simulink model "Cartpole_simulink"  (R2023a)
settings: Solver=FixedStepAuto  StartTime=0.0  StopTime=20  FixedStep=0.1  RelTol=1e-3
settings Model: Creator=rohan  LastModifiedBy=harsh
settings OptimizationCC: ReuseModelBlockBuffer=off

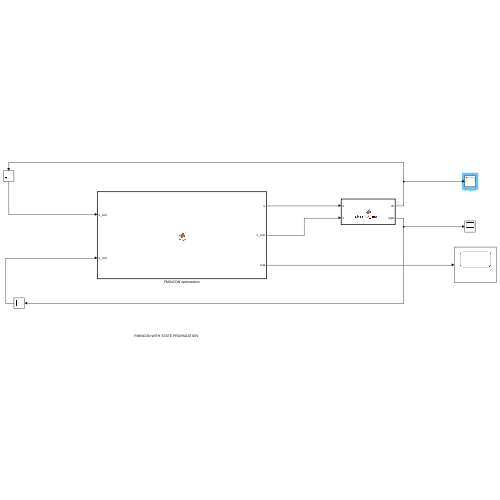
[thumbnail: Simulink's stored preview of the top-level diagram]
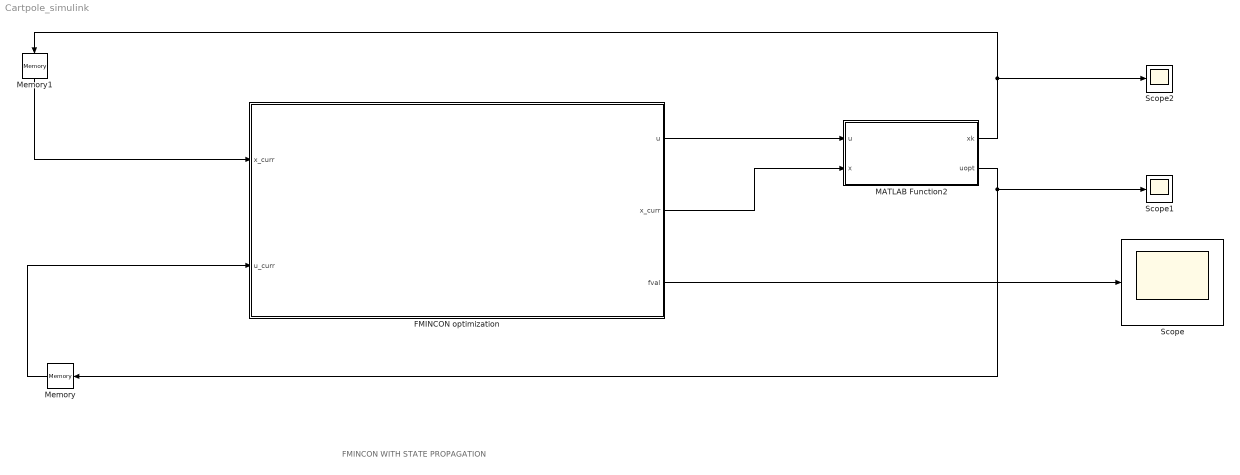
== system Cartpole_simulink ==
  note: FMINCON WITH STATE PROPAGATION
  FMINCON optimization : MATLAB Function  TreatAsAtomicUnit=on
  MATLAB Function2 : MATLAB Function  TreatAsAtomicUnit=on
  Memory : Memory  InitialCondition=zeros(10,1)
  Memory1 : Memory  InitialCondition=[0;0;-pi;0]
  Scope : Scope
  Scope1 : Scope
  Scope2 : Scope
  wires:
  FMINCON optimization/3(fval) -> Scope/1
  Memory/1 -> FMINCON optimization/2(u_curr)
  Memory1/1 -> FMINCON optimization/1("x_curr ")
  FMINCON optimization/1(u) -> MATLAB Function2/1(u)
  FMINCON optimization/2(x_curr) -> MATLAB Function2/2(x)
  MATLAB Function2/1(xk) -> Scope2/1, Memory1/1
  MATLAB Function2/2(uopt) -> Scope1/1, Memory/1

== matlab function Cartpole_simulink/FMINCON optimization ==
  data: u output; x_curr output; fval output; x_curr input; u_curr input
function [u, x_curr, fval] = mpc(x_curr, u_curr)
  N = 10;
  x = zeros(4,1);
  u = zeros(N,1);
  fval = 0;

  coder.extrinsic('Cartpole_mpc_function'); % <- Informing the Coder
  
  % Calling fmincon
  [u, fval] = Cartpole_mpc_function(x_curr,u_curr); % <- Optimal problem wrapper call
  disp("check")
end

== matlab function Cartpole_simulink/MATLAB Function2 ==
  data: u input; x input; xk output; uopt output
function [xk, uopt] = discrete_model(u,x)
    Ts=0.1;
    M=10;
    delta = Ts/M;
    xk=x;
    for ct=1:M
        xk = xk + delta*Continuous_model(xk,u);
    end
    uopt = u;
end

function dxdt = Continuous_model(x, u)
 mCart = 1;  % cart mass
 mPend = 1;  % pendulum mass
 g = 9.81;   % gravity of earth
 L = 0.5;    % pendulum length
 Kd = 10;    % cart damping
 %% Obtain x, u and y
 % x
 z_dot = x(2);
 theta = x(3);
 theta_dot = x(4);
 % u
 F = u(1);
 %% Compute dxdt
 dxdt = x;
 % z_dot
 dxdt(1) = z_dot;
 % z_dot_dot
 dxdt(2) = (F - Kd*z_dot - mPend*L*theta_dot^2*sin(theta) + mPend*g*sin(theta)*cos(theta)) / (mCart + mPend*sin(theta)^2);
 % theta_dot
 dxdt(3) = theta_dot;
 % theta_dot_dot
 dxdt(4) = ((F - Kd*z_dot - mPend*L*theta_dot^2*sin(theta))*cos(theta)/(mCart + mPend) + g*sin(theta)) / (L - mPend*L*cos(theta)^2/(mCart + mPend));
end
